simulink model "turing"  (R2021a)
settings: Solver=VariableStepAuto  StartTime=0.0  StopTime=100  RelTol=1e-3
values from neighbouring files (symbols this model uses):
  eta = 0.85    [PIturing.m]    (also in XSteam.m = h / 3000; XSteam_h_ps.m = h / 3000; full_plant.m = 0.809489; full_plant_20.m = 0.809489)
  h_sg_out = XSteam('hV_T', T_sg_out)    [turbing_parameter_calculation.m]
  J = 8500    [PIturing.m]    (also in full_plant.m; full_plant_20.m; policy.m; reactor_core.m)
  Ndes = 3600    [PIturing.m]    (also in full_plant.m; full_plant_20.m; policy.m; reactor_core.m)
  Pc = 0.008    [PIturing.m]    (also in full_plant.m; full_plant_20.m; policy.m; reactor_core.m)
  Pg0 = 819    [PIturing.m]    (also in full_plant.m = Pt0; full_plant_20.m = Pt0; policy.m = Pt0; reactor_core.m = Pt0)
  s_sg = 5.86    [PIturing.m]    (also in full_plant.m = XSteam('sV_p', P_sg0*10); full_plant_20.m = XSteam('sV_p', P_sg0 * 10); policy.m = XSteam('sV_p', P_sg0*10); reactor_core.m = XSteam('sV_p', P_sg0*10))
  W = 680.4    [turbing_parameter_calculation.m]
settings Model: Creator=xxc90  LastModifiedBy=xxc90

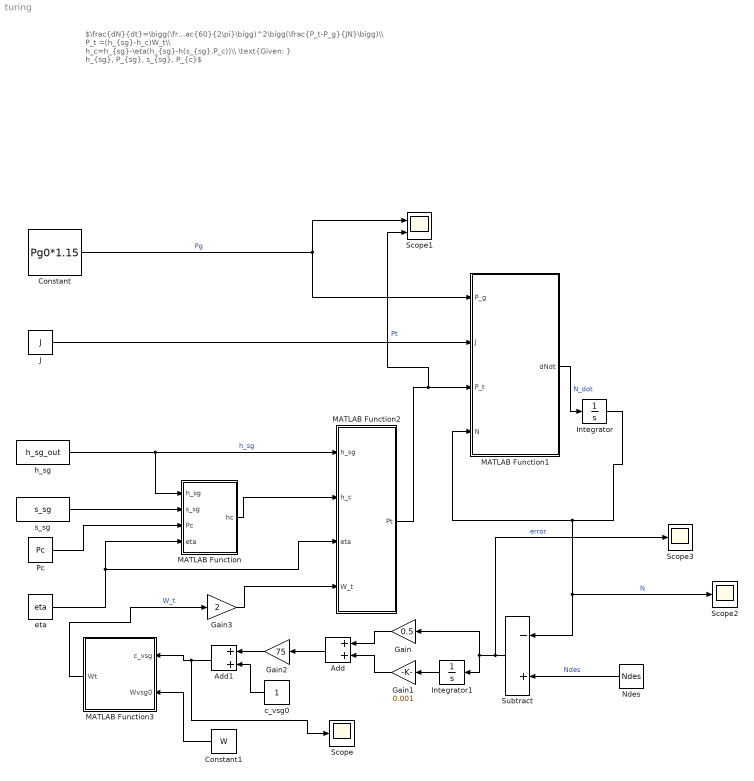
== system turing ==
  note: $\frac{dN}{dt}=\bigg(\frac{60}{2\pi}\bigg)^2\bigg(\frac{P_t-P_g}{JN}\bigg)\\ P_t =(h_{sg}-h_c)W_t\\ h_c=h_{sg}-\eta(h_{sg}-h(s_{sg},P_c))\\ \text{Given: } h_{sg}, P_{sg}, s_{sg}, P_{c}$
  Add : Sum
  Add1 : Sum
  Constant : Constant  Value=Pg0*1.15
  Constant1 : Constant  Value=W
  Gain : Gain  Gain=0.5
  Gain1 : Gain  Gain=0.001
  Gain2 : Gain  Gain=75
  Gain3 : Gain  Gain=2
  Integrator : Integrator  InitialCondition=3600
  Integrator1 : Integrator
  J : Constant  Value=J
  MATLAB Function : MATLAB Function  TreatAsAtomicUnit=on
  MATLAB Function1 : MATLAB Function  TreatAsAtomicUnit=on
  MATLAB Function2 : MATLAB Function  TreatAsAtomicUnit=on
  MATLAB Function3 : MATLAB Function  TreatAsAtomicUnit=on
  Ndes : Constant  Value=Ndes
  Pc : Constant  Value=Pc
  Scope : Scope
  Scope1 : Scope  NumInputPorts=2
  Scope2 : Scope
  Scope3 : Scope
  Subtract : Sum  Inputs=-+
  c_vsg0 : Constant
  eta : Constant  Value=eta
  h_sg : Constant  Value=h_sg_out
  s_sg : Constant  Value=s_sg
  wires:
  MATLAB Function1/1(dNdt) -> Integrator/1  "N_dot"
  Integrator/1 -> MATLAB Function1/4(N), Scope2/1, Subtract/1  "N"
  MATLAB Function2/1(Pt) -> Scope1/2, MATLAB Function1/3(P_t)  "Pt"
  h_sg/1 -> MATLAB Function/1(h_sg), MATLAB Function2/1(h_sg)  "h_sg"
  s_sg/1 -> MATLAB Function/2(s_sg)
  Ndes/1 -> Subtract/2  "Ndes"
  Subtract/1 -> Scope3/1, Gain/1, Integrator1/1  "error"
  Integrator1/1 -> Gain1/1
  Gain/1 -> Add/1
  Gain1/1 -> Add/2
  Add/1 -> Gain2/1
  Constant/1 -> MATLAB Function1/1(P_g), Scope1/1  "Pg"
  eta/1 -> MATLAB Function/4(eta), MATLAB Function2/3(eta)
  MATLAB Function/1(hc) -> MATLAB Function2/2(h_c)
  Pc/1 -> MATLAB Function/3(Pc)
  J/1 -> MATLAB Function1/2(J)
  Gain3/1 -> MATLAB Function2/4(W_t)
  MATLAB Function3/1(Wt) -> Gain3/1  "W_t"
  Constant1/1 -> MATLAB Function3/2(Wvsg0)
  Gain2/1 -> Add1/1
  c_vsg0/1 -> Add1/2
  Add1/1 -> Scope/1, MATLAB Function3/1(c_vsg)

== matlab function turing/MATLAB Function1 ==
  data: P_g input; J input; dNdt output; P_t input; N input
function dNdt = dNdt(P_g, J, P_t, N)
    dNdt = (60 / (2*pi))^2 * (P_t - P_g) / (J*N);
end

== matlab function turing/MATLAB Function ==
  data: h_sg input; s_sg input; Pc input; hc output; eta input
function hc = hc(h_sg,  s_sg, Pc, eta)
    hc = 0;
    fun = 'h_ps';
    hc = h_sg - eta * (h_sg - XSteam_h_ps(fun, Pc*10, s_sg));
end

== matlab function turing/MATLAB Function2 ==
  data: h_sg input; Pt output; h_c input; eta input; W_t input
function Pt = Pt(h_sg, h_c, eta, W_t)
    Pt = (h_sg - h_c) * W_t * eta / 1000;
end

== matlab function turing/MATLAB Function3 ==
  data: c_vsg input; Wvsg0 input; Wt output
function Wt = Wt(c_vsg, Wvsg0)
    Wt = Wvsg0 * c_vsg;
end
